simulink model "myScenario3MPC"  (R2019b)
settings: Solver=FixedStepAuto  StartTime=0.0  StopTime=100  RelTol=1e-3
model workspace (MAT data in the model file):
  firstWarning = 1
  originalScenarioChecksum = 'A7FFDCFCB80878E927950BD42491A1A0'
values from neighbouring files (symbols this model uses):
  driver_I = 0.1    [myACCSetUp.m]    (also in myACCSetUp2.m; myACCSetUp3.m; myACCSetUp3MPC.m)
  driver_P = 0.2    [myACCSetUp.m]    (also in myACCSetUp2.m; myACCSetUp3.m; myACCSetUp3MPC.m)
  lr = 1.6    [myACCSetUp.m]    (also in myACCSetUp2.m; myACCSetUp3.m; myACCSetUp3MPC.m)
  M = 2    [myACCSetUp.m]    (also in myACCSetUp2.m; myACCSetUp3.m; myACCSetUp3MPC.m)
  m = 1575    [myACCSetUp.m]    (also in myACCSetUp2.m; myACCSetUp3.m; myACCSetUp3MPC.m)
  N = 3    [myACCSetUp.m]    (also in myACCSetUp2.m; myACCSetUp3.m; myACCSetUp3MPC.m)
  posSelector = [1,0,0,0,0,0; 0,0,1,0,0,0]    [myACCSetUp.m]    (also in myACCSetUp2.m; myACCSetUp3.m; myACCSetUp3MPC.m)
  R = 10^10    (= 10000000000)    [myACCSetUp.m]    (also in myACCSetUp2.m = 760000000; myACCSetUp3.m; myACCSetUp3MPC.m)
  tau = 0.5    [myACCSetUp.m]    (also in myACCSetUp2.m; myACCSetUp3.m; myACCSetUp3MPC.m)
  time_gap = 1.5    [myACCSetUp.m]    (also in myACCSetUp2.m; myACCSetUp3.m; myACCSetUp3MPC.m)
  Ts = 0.1    [myACCSetUp.m]    (also in myACCSetUp2.m; myACCSetUp3.m; myACCSetUp3MPC.m)
  v_set = 21.5    [myACCSetUp.m]    (also in myACCSetUp2.m; myACCSetUp3.m = 30; myACCSetUp3MPC.m = 30)
  yawerr_gain = 2    [myACCSetUp.m]    (also in myACCSetUp2.m; myACCSetUp3.m; myACCSetUp3MPC.m)
undefined symbols (not defined in the file or in its folder): driving
libraries: drivingscenarioandsensors x3, drivinglib x2, mpcadaslib x1, simulink x1, autolibshared x1
settings Model: Creator=Administrator  LastModifiedBy=Administrator

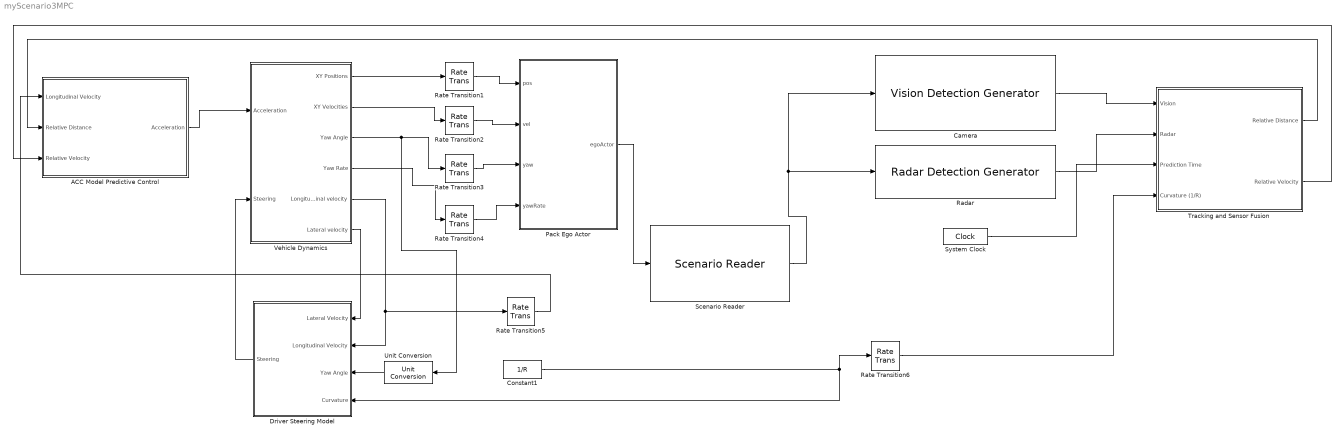
== system myScenario3MPC ==
  ACC Model Predictive Control : Subsystem  TreatAsAtomicUnit=on  VariantControl=controller_type == 2
      settings: RTWFileNameOpts=Use function name
  Camera : drivingscenarioandsensors/Vision Detection Generator  SensorIndex=1  DetectorOutput=Objects only  UpdateInterval=0.1  LaneUpdateInterval=0.1  SensorLocation=[3.7 0]  Height=1.1  Yaw=0  Pitch=1  Roll=0  BusNameSource=Property  BusName=BusVision  BusName2Source=Auto  BusName2=BusLaneDetections  MaxNumDetectionsSource=Property  MaxNumDetections=20  MaxNumLanesSource=Property  MaxNumLanes=30  DetectionCoordinates=Ego Cartesian  SimulateUsing=Interpreted execution  MaxRange=150  BoundingBoxAccuracy=5  ProcessNoiseIntensity=5  MaxSpeed=50  MaxAllowedOcclusion=0.5  MinObjectImageSize=[15 15]  DetectionProbability=0.9  FalsePositivesPerImage=0.1  MinLaneImageSize=[20 3]  LaneBoundaryAccuracy=3  HasNoise=on  InitialSeedSource=Repeatable  InitialSeed=0  UsedSeed=0  ActorProfilesSource=Parameters  ActorProfilesParameters=driving.internal.ActorProfilesParameters  ActorProfilesExpression=[struct('ActorID',1,'ClassID',1,'Length',4.7,'Width',1.8,'Height',1.4,'OriginOffset',[-1.35 0 0],'RCSPattern',[10 10;10 10],'RCSAzimuthAngles',[-180 180],'RCSElevationAngles',[-90 90]); struct('ActorID',2,'ClassID',1,'Length',4.7,'Width',1.8,'Height',1.4,'OriginOffset',[-1.35 0 0],'RCSPattern',[10 10;10 10],'RCSAzimuthAngles',[-180 180],'RCSElevationAngles',[-90 90])]  Intrinsics=driving.internal.cameraIntrinsics('FocalLength',[ 800, 800 ],'PrincipalPoint',[320 240],'ImageSize',[480 640],'RadialDistortion',[0 0],'TangentialDistortion',[0 0],'Skew',0)
      settings: SourceProductName=Automated Driving Toolbox
  Constant1 : Constant  Value=1/R
  Driver Steering Model : Subsystem
  Pack Ego Actor : MATLAB Function  TreatAsAtomicUnit=on
  Radar : drivingscenarioandsensors/Radar Detection Generator  SensorIndex=2  UpdateInterval=0.1  SensorLocation=[3.7 0]  Height=0.2  Yaw=0  Pitch=0  Roll=0  BusNameSource=Property  BusName=BusRadar  MaxNumDetectionsSource=Property  MaxNumDetections=50  DetectionCoordinates=Ego Cartesian  SimulateUsing=Interpreted execution  AzimuthResolution=4  ElevationResolution=10  RangeResolution=2.5  RangeRateResolution=0.5  AzimuthBiasFraction=0.1  ElevationBiasFraction=0.1  RangeBiasFraction=0.05  RangeRateBiasFraction=0.05  FieldOfView=[20 5]  MaxRange=180  RangeRateLimits=[-100 100]  DetectionProbability=0.9  FalseAlarmRate=1e-06  ReferenceRange=100  ReferenceRCS=0  HasElevation=off  HasRangeRate=on  HasNoise=on  HasFalseAlarms=on  HasOcclusion=on  InitialSeedSource=Repeatable  InitialSeed=0  UsedSeed=0  ActorProfilesSource=Parameters  ActorProfilesParameters=driving.internal.ActorProfilesRadarParameters  ActorProfilesExpression=[struct('ActorID',1,'ClassID',1,'Length',4.7,'Width',1.8,'Height',1.4,'OriginOffset',[-1.35 0 0],'RCSPattern',[10 10;10 10],'RCSAzimuthAngles',[-180 180],'RCSElevationAngles',[-90 90]); struct('ActorID',2,'ClassID',1,'Length',4.7,'Width',1.8,'Height',1.4,'OriginOffset',[-1.35 0 0],'RCSPattern',[10 10;10 10],'RCSAzimuthAngles',[-180 180],'RCSElevationAngles',[-90 90])]
      settings: SourceProductName=Automated Driving Toolbox  SourceProductBaseCode=DR
  Rate Transition{1..6} (6 alike) : RateTransition  OutPortSampleTime=Ts
  Scenario Reader : drivingscenarioandsensors/Scenario Reader  ScenarioSource=From file  ScenarioFileName=E:\GITHUB\matlabAutoDriving\DrivingSimulation\myScenario4.mat  ScenarioVariableName=scenario  OutputCoordinateSystem=Vehicle coordinates  EgoVehicleSource=Input port  EgoVehicleActorID=1  SampleTime=0.1  LaneBoundaryOutput=None  LaneBoundaryDistance=0:0.5:9.5  LaneBoundaryLocation=Center of lane markings  BusNameSource=Property  BusName=BusActors1  BusName2Source=Auto  BusName2=BusLaneBoundaries  SimulateUsing=Interpreted execution
      settings: SourceProductName=Automated Driving Toolbox
  System Clock : DigitalClock  SampleTime=Ts
  Tracking and Sensor Fusion : Subsystem  TreatAsAtomicUnit=on
      settings: RTWFileNameOpts=Use function name
  Unit Conversion : UnitConversion
  Vehicle Dynamics : Subsystem  VariantControl=Variant2
  wires:
  Rate Transition1/1 -> Pack Ego Actor/1(pos)
  Rate Transition2/1 -> Pack Ego Actor/2(vel)
  Rate Transition3/1 -> Pack Ego Actor/3(yaw)
  Vehicle Dynamics/1(XY Positions) -> Rate Transition1/1
  Vehicle Dynamics/2(XY Velocities) -> Rate Transition2/1
  Vehicle Dynamics/3(Yaw Angle) -> Unit Conversion/1, Rate Transition3/1
  Vehicle Dynamics/4(Yaw Rate) -> Rate Transition4/1
  Tracking and Sensor Fusion/1(Relative Distance) -> ACC Model Predictive Control/2(Relative Distance)
  Tracking and Sensor Fusion/2(Relative Velocity) -> ACC Model Predictive Control/3(Relative Velocity)
  System Clock/1 -> Tracking and Sensor Fusion/3(Prediction Time)
  Constant1/1 -> Driver Steering Model/4(Curvature), Rate Transition6/1
  Driver Steering Model/1(Steering) -> Vehicle Dynamics/2(Steering)
  Vehicle Dynamics/6(Lateral velocity) -> Driver Steering Model/1(Lateral Velocity)
  Vehicle Dynamics/5(Longitudinal velocity) -> Rate Transition5/1, Driver Steering Model/2(Longitudinal Velocity)
  Unit Conversion/1 -> Driver Steering Model/3(Yaw Angle)
  Rate Transition6/1 -> Tracking and Sensor Fusion/4(Curvature (1/R))
  Rate Transition5/1 -> ACC Model Predictive Control/1(Longitudinal Velocity)
  Pack Ego Actor/1(egoActor) -> Scenario Reader/1
  Scenario Reader/1 -> Camera/1, Radar/1
  Camera/1 -> Tracking and Sensor Fusion/1(Vision)
  Radar/1 -> Tracking and Sensor Fusion/2(Radar)
  Rate Transition4/1 -> Pack Ego Actor/4(yawRate)
  ACC Model Predictive Control/1(Acceleration) -> Vehicle Dynamics/1(Acceleration)

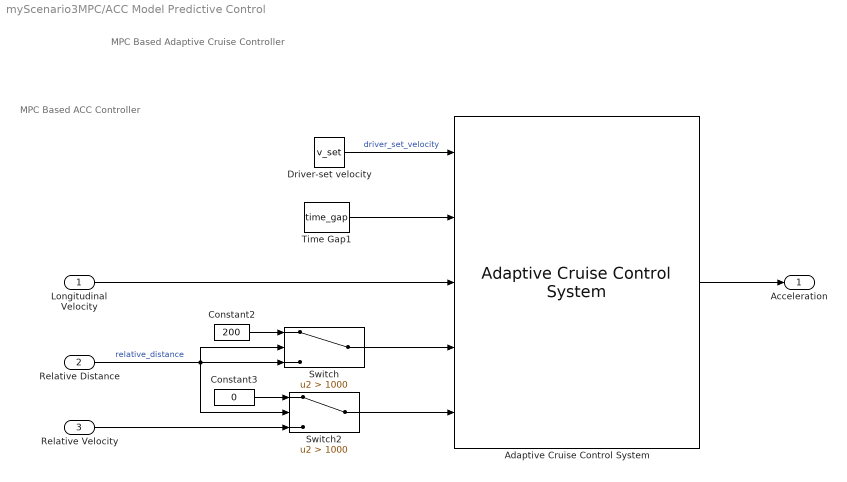
== system myScenario3MPC/ACC Model Predictive Control ==
  note: MPC Based Adaptive Cruise Controller
  note: MPC Based ACC Controller
  Longitudinal Velocity : Inport
  Relative Distance : Inport  Port=2
  Relative Velocity : Inport  Port=3
  Adaptive Cruise Control System : mpcadaslib/Adaptive Cruise Control System  EgoModel=G  InitialEgoVelocity=v0_ego  DefaultSpacing=default_spacing  MaxVelocity=50  MinAcceleration=min_ac  amin_ext=off  MaxAcceleration=max_ac  amax_ext=off  Ts=Ts  PredictionHorizon=30  ControllerBehavior=0.5  suboptimal=off  maxiter=10  datatypeopt=double  optmode=off  trackmode=off
      settings: SourceProductName=Model Predictive Control Toolbox
  Constant2 : Constant  Value=200  SampleTime=Ts
  Constant3 : Constant  Value=0  SampleTime=Ts
  Driver-set velocity : Constant  Value=v_set  SampleTime=Ts
  Switch : Switch  Criteria=u2 > Threshold  Threshold=1000
  Switch2 : Switch  Criteria=u2 > Threshold  Threshold=1000
  Time Gap1 : Constant  Value=time_gap  SampleTime=Ts
  Acceleration : Outport  OutDataTypeStr=double  PortDimensions=1  SampleTime=[0.10000000000000001,0]  VectorParamsAs1DForOutWhenUnconnected=off
  wires:
  Adaptive Cruise Control System/1 -> Acceleration/1
  Driver-set velocity/1 -> Adaptive Cruise Control System/1  "driver_set_velocity"
  Constant2/1 -> Switch/1
  Relative Distance/1 -> Switch/3, Switch2/2, Switch/2  "relative_distance"
  Constant3/1 -> Switch2/1
  Relative Velocity/1 -> Switch2/3
  Time Gap1/1 -> Adaptive Cruise Control System/2
  Longitudinal Velocity/1 -> Adaptive Cruise Control System/3
  Switch/1 -> Adaptive Cruise Control System/4
  Switch2/1 -> Adaptive Cruise Control System/5

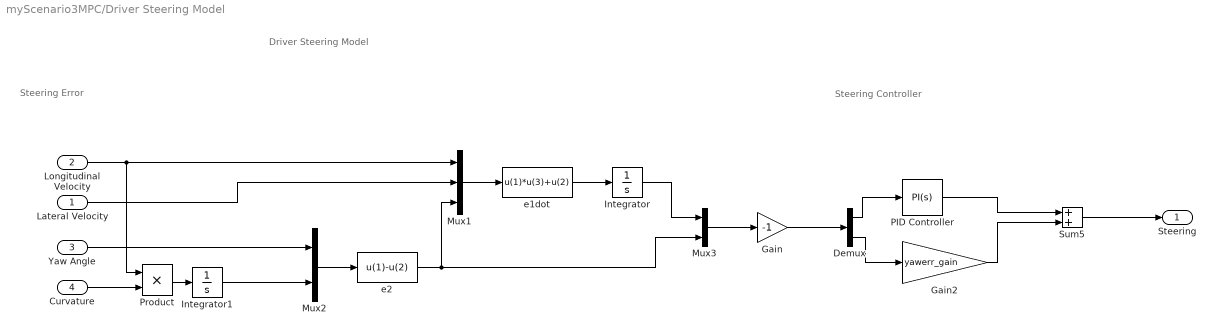
== system myScenario3MPC/Driver Steering Model ==
  note: Steering Controller
  note: Steering Error
  note: Driver Steering Model
  Lateral Velocity : Inport
  Longitudinal Velocity : Inport  Port=2
  Yaw Angle : Inport  Port=3  Unit=rad
  Curvature : Inport  Port=4
  Demux : Demux  Outputs=2
  Gain : Gain  Gain=-1
  Gain2 : Gain  Gain=yawerr_gain
  Integrator : Integrator
  Integrator1 : Integrator
  Mux1 : Mux  Inputs=3
  Mux2 : Mux  Inputs=2
  Mux3 : Mux  Inputs=2
  PID Controller : simulink/Continuous/PID Controller  Controller=PI  Form=Parallel  TimeDomain=Continuous-time  SampleTime=-1  IntegratorMethod=Forward Euler  FilterMethod=Forward Euler  ControllerParametersSource=internal  P=driver_P  I=driver_I  D=0  UseFilter=on  N=100  TunerSelectOption=Transfer Function Based (PID Tuner App)  InitialConditionSource=internal  InitialConditionForIntegrator=0  InitialConditionForFilter=0  DifferentiatorICPrevScaledInput=0  ExternalReset=none  TrackingMode=off  Kt=1  LimitOutput=off  UpperSaturationLimit=inf  LowerSaturationLimit=-inf  LinearizeAsGain=on  AntiWindupMode=none  Kb=1  POutMin=[]  POutMax=[]  IOutMin=[]  IOutMax=[]  DOutMin=[]  DOutMax=[]  NOutMin=[]  NOutMax=[]  SumOutMin=[]  SumOutMax=[]  SaturationOutMin=[]  SaturationOutMax=[]  PParamMin=[]  PParamMax=[]  IParamMin=[]  IParamMax=[]  DParamMin=[]  DParamMax=[]  NParamMin=[]  NParamMax=[]  KbParamMin=[]  KbParamMax=[]  KtParamMin=[]  KtParamMax=[]  KbOutMin=[]  KbOutMax=[]  KtOutMin=[]  KtOutMax=[]  IntegratorOutMin=[]  IntegratorOutMax=[]  FilterOutMin=[]  FilterOutMax=[]  SumI1OutMin=[]  SumI1OutMax=[]  SumI2OutMin=[]  SumI2OutMax=[]  SumI3OutMin=[]  SumI3OutMax=[]  SumI4OutMin=[]  SumI4OutMax=[]  SumDOutMin=[]  SumDOutMax=[]  DifferentiatorOutMin=[]  DifferentiatorOutMax=[]  FilterDiffOutCoefMin=[]  FilterDiffOutCoefMax=[]  ReciprocalOutMin=[]  ReciprocalOutMax=[]  SumDenOutMin=[]  SumDenOutMax=[]  SumNumOutMin=[]  SumNumOutMax=[]  DivideOutMin=[]  DivideOutMax=[]  IntegratorContinuousStateAttributes=''  IntegratorStateMustResolveToSignalObject=off  IntegratorRTWStateStorageClass=Auto  FilterContinuousStateAttributes=''  FilterStateMustResolveToSignalObject=off  FilterRTWStateStorageClass=Auto  ParallelPVariant=InternalParameters  IdealPVariant=Disabled  IVariant=InternalParameters  DVariant=Disabled  IntegratorVariant=Continuous  SatVariant=Disabled  AWVariant=Passthrough  PCopyVariant=Disabled  TRVariant=Disabled  FdbkBlocksVariant=Forward  IdealPFdbkVariant=Disabled  SatFdbkVariant=Disabled  DerivativeFilterVariant=Disabled  NVariant=Disabled  NCopyVariant=Disabled_SignalSpec  FilterICVariant=Disabled  IntegratorICVariant=InternalICs  ExternalResetVariant=Disabled  TRSumVariant=Passthrough  SumFdbkVariant=Disabled  SumVariant=Sum_PI
  Product : Product
  Sum5 : Sum
  e1dot : Fcn  Expr=u(1)*u(3)+u(2)
  e2 : Fcn  Expr=u(1)-u(2)
  Steering : Outport  VectorParamsAs1DForOutWhenUnconnected=off
  wires:
  e1dot/1 -> Integrator/1
  Mux2/1 -> e2/1
  e2/1 -> Mux1/3, Mux3/2
  Mux3/1 -> Gain/1
  Lateral Velocity/1 -> Mux1/2
  Yaw Angle/1 -> Mux2/1
  Mux1/1 -> e1dot/1
  Integrator/1 -> Mux3/1
  Product/1 -> Integrator1/1
  Integrator1/1 -> Mux2/2
  Curvature/1 -> Product/2
  Longitudinal Velocity/1 -> Product/1, Mux1/1
  Gain2/1 -> Sum5/2
  PID Controller/1 -> Sum5/1
  Demux/2 -> Gain2/1
  Sum5/1 -> Steering/1
  Demux/1 -> PID Controller/1
  Gain/1 -> Demux/1

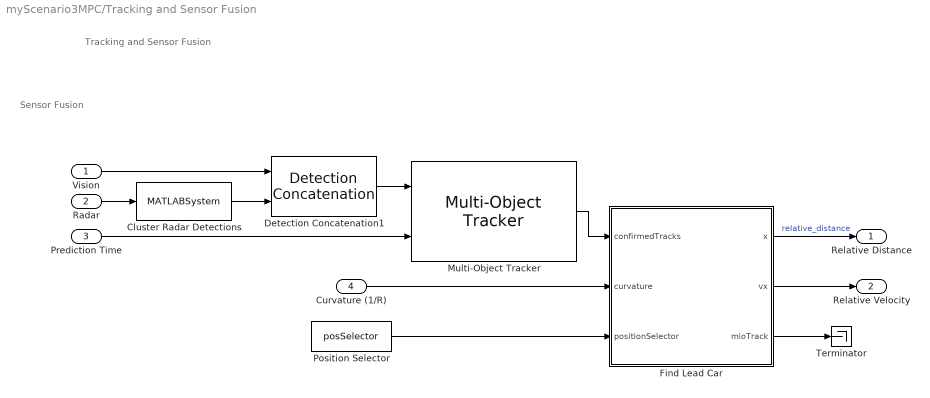
== system myScenario3MPC/Tracking and Sensor Fusion ==
  note: Sensor Fusion
  note: Tracking and Sensor Fusion
  Vision : Inport  OutDataTypeStr=Bus: BusVision  PortDimensions=[1 1]  SampleTime=[0.10000000000000001,0]  BusOutputAsStruct=on
  Radar : Inport  Port=2  OutDataTypeStr=Bus: BusRadar  PortDimensions=[1 1]  SampleTime=[0.10000000000000001,0]  BusOutputAsStruct=on
  Prediction Time : Inport  Port=3  OutDataTypeStr=double  PortDimensions=[1 1]  SampleTime=[0.10000000000000001,0]  BusOutputAsStruct=on
  Curvature (1/R) : Inport  Port=4  OutDataTypeStr=double  PortDimensions=[1 1]  SampleTime=[0.10000000000000001,0]  BusOutputAsStruct=on
  Cluster Radar Detections : MATLABSystem  System=helperClusterDetections  ClusterSize=clusterSize  BusNameSource=Auto  BusName=BusClusterDetections  SimulateUsing=Interpreted execution
      mask Type: helperClusterDetections
      mask Display:
      | disp(['Detection' char(10) 'Clustering']);
      | port_label('input',1,'In');
      | port_label('output',1,'Out');
  Detection Concatenation1 : drivinglib/Detection Concatenation  NumInputs=2  BusNameSource=Auto  BusName=BusDetectionConcatenation1  SimulateUsing=Interpreted execution
      settings: SourceProductName=Automated Driving Toolbox  SourceProductBaseCode=DR
  Find Lead Car : MATLAB Function  TreatAsAtomicUnit=on
  Multi-Object Tracker : drivinglib/Multi-Object Tracker  FilterInitializationFcn=initcvekf  AssignmentThreshold=assigThresh  ConfirmationParameters=[M,N]  NumCoastingUpdates=numCoasts  MaxNumTracks=numTracks  MaxNumSensors=numSensors  TimeInputSource=Input port  HasCostMatrixInput=off  BusNameSource=Property  BusName=BusMultiObjectTracker1  TentativeTracksOutputPort=off  AllTracksOutputPort=off  SimulateUsing=Interpreted execution
      settings: SourceProductName=Automated Driving Toolbox  SourceProductBaseCode=DR
  Position Selector : Constant  Value=posSelector
  Terminator : Terminator
  Relative Distance : Outport  VectorParamsAs1DForOutWhenUnconnected=off
  Relative Velocity : Outport  Port=2  VectorParamsAs1DForOutWhenUnconnected=off
  wires:
  Cluster Radar Detections/1 -> Detection Concatenation1/2
  Vision/1 -> Detection Concatenation1/1
  Prediction Time/1 -> Multi-Object Tracker/2
  Find Lead Car/2(vx) -> Relative Velocity/1
  Radar/1 -> Cluster Radar Detections/1
  Curvature (1/R)/1 -> Find Lead Car/2(curvature)
  Multi-Object Tracker/1 -> Find Lead Car/1(confirmedTracks)
  Detection Concatenation1/1 -> Multi-Object Tracker/1
  Find Lead Car/1(x) -> Relative Distance/1  "relative_distance"
  Position Selector/1 -> Find Lead Car/3(positionSelector)
  Find Lead Car/3(mioTrack) -> Terminator/1

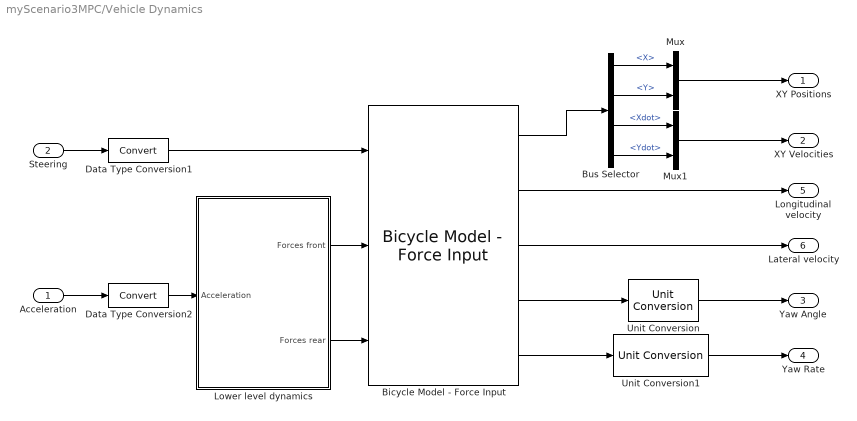
== system myScenario3MPC/Vehicle Dynamics ==
  Acceleration : Inport  Unit=m/s^2
  Steering : Inport  Port=2  Unit=rad
  Bicycle Model - Force Input : autolibshared/Bicycle Model - Force Input  trackMode=Single (bicycle)  inputMode=External longitudinal forces  frontSteerMode=on  rearSteerMode=off  windMode=off  muMode=off  extFMode=off  extMMode=off  aMode=3  NF=2  NR=2  m=m  a=lf  b=lr  h=0.35  X_o=x0_ego  xdot_o=v0_ego  CalphaMode=off  sigmaMode=on  w=[1.4,1.4]  Cy_f=Cf  Cy_r=Cr  sigma_f=.1  sigma_r=.1  alpha_f_brk=[-.1 .1]  Cy_f_data=[-9e3 9e3]  alpha_r_brk=[-.1 .1]  Cy_r_data=[-9e3 9e3]  Y_o=y0_ego  ydot_o=0  Izz=Iz  psi_o=0  r_o=0  Af=0  Cd=.3  Cl=.1  Cpm=.1  beta_w=[0:0.01:0.3]  Cs=[0:0.03:0.9]  Cym=[0:0.01:0.3]  Pabs=101325  Tair=273  g=9.81  mu=1  xdot_tol=.01  Fznom=5000  Fxtire_sat=1e6  Fytire_sat=1e6  longOff=0  latOff=0  vertOff=0
      settings: SourceProductName=Powertrain Blockset  SourceProductBaseCode=PW
  Bus Selector : BusSelector  OutputSignals=InertFrm.FrntAxl.Disp.X,InertFrm.FrntAxl.Disp.Y,InertFrm.FrntAxl.Vel.Xdot,InertFrm.FrntAxl.Vel.Ydot
  Data Type Conversion1 : DataTypeConversion
  Data Type Conversion2 : DataTypeConversion
  Lower level dynamics : Subsystem
  Mux : Mux  Inputs=2
  Mux1 : Mux  Inputs=2
  Unit Conversion : UnitConversion
  Unit Conversion1 : UnitConversion
  XY Positions : Outport  Unit=m  VectorParamsAs1DForOutWhenUnconnected=off
  XY Velocities : Outport  Port=2  Unit=m/s  VectorParamsAs1DForOutWhenUnconnected=off
  Yaw Angle : Outport  Port=3  Unit=deg  VectorParamsAs1DForOutWhenUnconnected=off
  Yaw Rate : Outport  Port=4  Unit=degree/s  VectorParamsAs1DForOutWhenUnconnected=off
  Longitudinal velocity : Outport  Port=5  VectorParamsAs1DForOutWhenUnconnected=off
  Lateral velocity : Outport  Port=6  VectorParamsAs1DForOutWhenUnconnected=off
  wires:
  Lower level dynamics/2(Forces rear) -> Bicycle Model - Force Input/3
  Lower level dynamics/1(Forces front) -> Bicycle Model - Force Input/2
  Data Type Conversion2/1 -> Lower level dynamics/1(Acceleration)
  Acceleration/1 -> Data Type Conversion2/1
  Steering/1 -> Data Type Conversion1/1
  Bus Selector/1 -> Mux/1  "<X>"
  Bicycle Model - Force Input/4 -> Unit Conversion/1
  Bus Selector/4 -> Mux1/2  "<Ydot>"
  Bus Selector/2 -> Mux/2  "<Y>"
  Bicycle Model - Force Input/2 -> Longitudinal velocity/1
  Bus Selector/3 -> Mux1/1  "<Xdot>"
  Bicycle Model - Force Input/1 -> Bus Selector/1
  Bicycle Model - Force Input/3 -> Lateral velocity/1
  Mux/1 -> XY Positions/1
  Mux1/1 -> XY Velocities/1
  Bicycle Model - Force Input/5 -> Unit Conversion1/1
  Data Type Conversion1/1 -> Bicycle Model - Force Input/1
  Unit Conversion/1 -> Yaw Angle/1
  Unit Conversion1/1 -> Yaw Rate/1

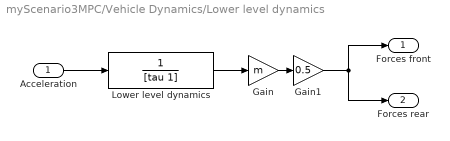
== system myScenario3MPC/Vehicle Dynamics/Lower level dynamics ==
  Acceleration : Inport
  Gain : Gain  Gain=m
  Gain1 : Gain  Gain=0.5
  Lower level dynamics : TransferFcn  Denominator=[tau 1]
  Forces front : Outport  VectorParamsAs1DForOutWhenUnconnected=off
  Forces rear : Outport  Port=2  VectorParamsAs1DForOutWhenUnconnected=off
  wires:
  Gain/1 -> Gain1/1
  Gain1/1 -> Forces front/1, Forces rear/1
  Acceleration/1 -> Lower level dynamics/1
  Lower level dynamics/1 -> Gain/1

== matlab function myScenario3MPC/Tracking and Sensor Fusion/Find Lead Car ==
  data: confirmedTracks input; x output double size=[1 1]; vx output size=[1 1]; curvature input; mioTrack output; positionSelector input
function [x,vx,mioTrack] = findLeadCar(confirmedTracks, curvature, positionSelector)
% This function finds the lead car: a car in front of the ego car that
% satisfies all the criteria below:
% * Within the ego car's lane.
% * In front of the ego car.
% * Closest to the ego car.

% Important notes:
% 1. If you change state definition, change the following:
%       State = [x;vx;y;vy;z;vz] (3D constant velocity)
numStates = 6;

% 2. The lane is defined using a parabolic model, where y=ax^2+bx+c. a is
%    equal to half the road curvature, b=0, and c is the offset of the lane
%    boundaries relative to the ego car. Overall lane width is assumed to
%    be 3.6m, typical highway lane width.
laneWidth = 3.6;

% 3. The ego car is assumed to be traveling in the middle of its lane, with
%    1.8m on each side of it. So, c=+1.8m for the left lane boundary and
%    -1.8m for the right lane boundary.
halfLaneWidth = laneWidth/2;

% Initialize outputs and parameters
maxX = cast(1000, 'like', confirmedTracks.Tracks(1).State);  % Far enough forward so that no track is expected to exceed this distance
trackID = 0;

for i = 1:confirmedTracks.NumTracks
    position = positionSelector * confirmedTracks.Tracks(i).State;
    x = position(1); % Longitudinal position of the track relative to ego
    y = position(2); % Lateral position of the track relative to ego
    
    if x < maxX && x > 0 % No point checking otherwise
        yleftLane  = polyval([curvature/2, 0,  halfLaneWidth],x); % Half a lane to the left
        yrightLane = polyval([curvature/2, 0, -halfLaneWidth],x); % Half a lane to the right
        
        % Find a new lead car
        if (yrightLane <= y) && (y <= yleftLane)
            maxX = x;
            trackID = i;
        end
    end
end

if trackID>0
    mioState = confirmedTracks.Tracks(trackID).State;
else
    mioState = inf(numStates,1,'like',confirmedTracks.Tracks(1).State);
end

% Output:
x = mioState(1);    % Longitudinal position of the lead car
vx = mioState(2);   % Longitudinal velocity of the lead car
mioTrack = trackID; % Index of the most important track

== matlab function myScenario3MPC/Pack Ego Actor ==
  data: pos input; vel input; yaw input; egoActor output Bus: BusActors1Actors size=1; yawRate input
function egoActor  = packEgo(pos,vel,yaw,yawRate)
% Pack ego information into a single ego actor bus
%
% Imoprtant note:
% Output is a bus of type BusActorsActors. This is the same bus used by the
% Scenario Reader to output an individual actor. If you change the
% output bus name of Scenario Reader, change the output bus name here
% as well by clicking on 'Edit Data' in the menu above.

egoActor = struct(...
    'ActorID',1,...
    'Position', [pos(1) pos(2) 0], ...
    'Velocity', [vel(1) vel(2) 0], ...
    'Roll', 0, ...
    'Pitch', 0, ...
    'Yaw', yaw, ...
    'AngularVelocity', [0 0 yawRate]);
